simulink model "base_sim"  (R2022a)
settings: Solver=VariableStepAuto  StartTime=0.0  StopTime=10.0  MaxStep=1e-2  RelTol=1e-3
undefined symbols (not defined in the file): a1, a2, B, dq0, dtheta0, K, m1, m2, q0, S, theta0
settings Model: Creator=mathe  LastModifiedBy=mathe

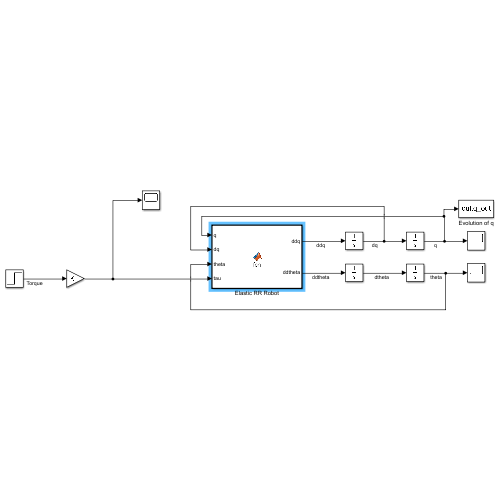
[thumbnail: Simulink's stored preview of the top-level diagram]
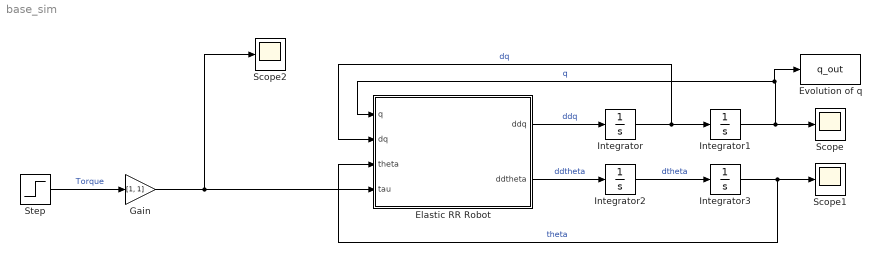
== system base_sim ==
  Elastic RR Robot : MATLAB Function  TreatAsAtomicUnit=on
  Evolution of q : ToWorkspace  VariableName=q_out  SaveFormat=Timeseries  SampleTime=-1
  Gain : Gain  Gain=[1, 1]
  Integrator : Integrator  InitialCondition=dq0
  Integrator1 : Integrator  InitialCondition=q0
  Integrator2 : Integrator  InitialCondition=dtheta0
  Integrator3 : Integrator  InitialCondition=theta0
  Scope : Scope
  Scope1 : Scope
  Scope2 : Scope
  Step : Step  SampleTime=0
  wires:
  Elastic RR Robot/1(ddq) -> Integrator/1  "ddq"
  Integrator/1 -> Integrator1/1, Elastic RR Robot/2(dq)  "dq"
  Integrator2/1 -> Integrator3/1  "dtheta"
  Elastic RR Robot/2(ddtheta) -> Integrator2/1  "ddtheta"
  Integrator3/1 -> Scope1/1, Elastic RR Robot/3(theta)  "theta"
  Integrator1/1 -> Elastic RR Robot/1(q), Evolution of q/1, Scope/1  "q"
  Step/1 -> Gain/1  "Torque"
  Gain/1 -> Scope2/1, Elastic RR Robot/4(tau)

== matlab function base_sim/Elastic RR Robot ==
  data: q input; ddq output; dq input; theta input; tau input; ddtheta output; K parameter; B parameter; m1 parameter; m2 parameter; a1 parameter; a2 parameter; S parameter
function [ddq, ddtheta] = fcn(q, dq, theta, tau, K, B, m1, m2, a1, a2, S)

% Compute dynamic matrices
[M, C, G] = dynamics(q, dq, m1, m2, a1, a2);

% State evolutions
ddq = M\(S.'*K*(theta - q) - C*dq - G);
ddtheta = B\(tau - K*(theta - q));
